simulink model "DBX_control_harness"  (R2015a)
settings: Solver=ode2  SolverMode=SingleTasking  StartTime=0.0  StopTime=inf  FixedStep=T_sim  RelTol=1e-3
values from neighbouring files (symbols this model uses):
  airport_alt = 587.5    [Run_DBX.m]
  latitude = 40.463650    (= 40.46365)    [Run_DBX.m]
  longitude = -3.554389    [Run_DBX.m]
  T_ctrl = 0.01    [Run_DBX.m]
  T_sim = 0.01    [Run_DBX.m]
undefined symbols (not defined in the file or in its folder): accel_sigmas, Alt_0, DBX_PWM, delta_a_L_0_servo, delta_a_R_0_servo, delta_rv_L_0_servo, delta_rv_R_0_servo, eta_1_0_servo, eta_2_0_servo, eta_3_0_servo, Euler_0, Euler_dot_sigmas, Euler_sigmas, g, GPS_pos_sig, Initial_Omegas, Newton, omgea_b_sigmas, qbar_sigma, quaternion_sigmas, Raphson, Roll_pich_sens, sigbuilder_block, Speed_sigmas, TAS_0, tau_1_0, tau_2_0, tau_3_0, Throtle_sens, Volt_noise, Yaw_sens
libraries: DBX_model x14, commnoisgen2 x9, simulink x3, powerlib_meascontrol x2, utility x1
(part 1 of 2)
settings Model: ExtModeTrigDuration=5000  Creator=DavidTorres  LastModifiedBy=david
settings DataIOCC: LimitDataPoints=off  SaveOutput=off  SignalLogging=off  DSMLogging=off  VisualizeSimOutput=off  SaveTime=off
settings OptimizationCC: InlineParams=on  UseDivisionForNetSlopeComputation=on  UseFloatMulNetSlope=on  InlineInvariantSignals=on  EnhancedBackFolding=on  EfficientFloat2IntCast=on  MaxStackSize=inf  SimCompilerOptimization=on
settings DebuggingCC: WriteAfterWriteMsg=EnableAllAsError  AlgebraicLoopMsg=error  ArtificialAlgebraicLoopMsg=error  SaveWithParameterizedLinksMsg=none  IntegerOverflowMsg=error  ParameterUnderflowMsg=error  ParameterTunabilityLossMsg=error  UniqueDataStoreMsg=error  AssertControl=DisableAll  StrictBusMsg=ErrorOnBusTreatedAsVector  NonBusSignalsTreatedAsBus=error  SFUnexpectedBacktrackingDiag=error  SFInvalidInputDataAccessInChartInitDiag=error  SFNoUnconditionalDefaultTransitionDiag=error  SFTransitionOutsideNaturalParentDiag=error  SFUnconditionalTransitionShadowingDiag=error  SFUndirectedBroadcastEventsDiag=error  SFTransitionActionBeforeConditionDiag=error  IntegerSaturationMsg=error
settings HardwareCC: ProdLargestAtomicInteger=Long  ProdLargestAtomicFloat=Float  ProdIntDivRoundTo=Zero  ProdEndianess=LittleEndian  ProdHWDeviceType=ARM Compatible->ARM 7  TargetUnknown=on
settings ModelReferenceCC: ModelReferenceNumInstancesAllowed=Single  ModelReferencePassRootInputsByReference=off

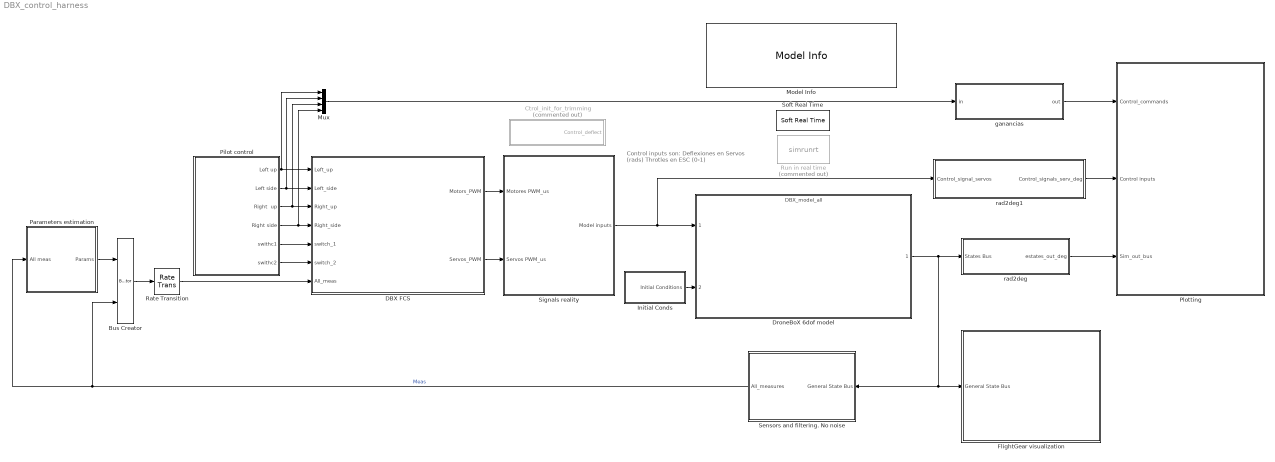
== system DBX_control_harness ==
  note: Control inputs son:
      | Deflexiones en Servos (rads)
      | Throtles en ESC (0-1)
  Bus Creator : BusCreator  Inputs=2
  Ctrol_init_for_trimming : Subsystem  Commented=on  TreatAsAtomicUnit=on
  DBX FCS : Subsystem
  DroneBoX 6dof model : ModelReference  ModelNameDialog=DBX_model_all.slx  SimulationMode=Normal  OverrideUsingVariant=Model_all  ModelReferenceVersion=1.02  CopyOfModelName=DBX_model_all.slx  DefaultDataLogging=on
      mask Display:
      | % % image('conv.jpg')
      | % %
      | % % port_label('output', 1, 'General State Bus')
      | % %
      | % % port_label('input', 1, 'Control Inputs')
      | % % port_label('input', 2, 'Initial Conditions')
      | % %
      | % %
      | % % % Variant dealing
      | % % ActiveVar = get_param(gcb,'activevariant');
      | % % disp(['{\bf\fontsize{16}',ActiveVar,'}'], 'texmode','on');
  FlightGear visualization : Subsystem  TreatAsAtomicUnit=on
      mask Display:
      | % % disp('{\bf\fontsize{20} Flight Gear}', 'texmode','on');
      | % % image('convFG.jpg')
      | % %
      | % % port_label('input', 1, 'General State Bus')
  Initial Conds : Subsystem  TreatAsAtomicUnit=on
  Model Info : simulink/Model-Wide Utilities/Model Info  Frame=on  DisplayStringWithTags=|  HorizontalTextAlignment=Center  LeftAlignmentValue=0.5  SourceBlockDiagram=DBX_control_harness  TagMaxNumber=20
      | Model %<ModelName>
      | 
      | Creado por %<Creator>
      | Modificado el %<LastModificationDate> por %<LastModifiedBy>
      | Version %<ModelVersion>
  Mux : Mux
  Parameters estimation : Subsystem  TreatAsAtomicUnit=on
  "Pilot control " : Subsystem  Variant=on  OverrideUsingVariant=Turnigy
  Plotting : Subsystem
      mask Display:
      | disp('{\bf\fontsize{20} Plotting}', 'texmode','on');
      | % port_label('input', 1, 'States')
      | % port_label('input', 2, 'Demans')
  Rate Transition : RateTransition  OutPortSampleTime=T_ctrl
  Run in real time : S-Function  Commented=on  FunctionName=simrunrt  Parameters=1
  Sensors and filtering. No noise : Subsystem  Variant=on  VariantControl=No noise  OverrideUsingVariant=Noise
  Signals reality : Subsystem
  Soft Real Time : utility/Soft Real Time  x=1
  ganancias : Subsystem
  rad2deg : Subsystem
  rad2deg1 : Subsystem
  wires:
  Initial Conds/1(Initial Conditions) -> DroneBoX 6dof model/2
  DroneBoX 6dof model/1 -> FlightGear visualization/1(General State Bus), Sensors and filtering. No noise/1(General State Bus), rad2deg/1(States Bus)
  rad2deg/1("estates_out_deg ") -> Plotting/3(Sim_out_bus)
  Signals reality/1(Model inputs) -> rad2deg1/1(Control_signal_servos), DroneBoX 6dof model/1
  Sensors and filtering. No noise/1(All_measures) -> Parameters estimation/1(All meas), Bus Creator/2  "Meas"
  Bus Creator/1 -> Rate Transition/1
  Parameters estimation/1(Params) -> Bus Creator/1
  DBX FCS/1(Motors_PWM) -> Signals reality/1(Motores PWM_us)
  DBX FCS/2(Servos_PWM) -> Signals reality/2(Servos PWM_us)
  Rate Transition/1 -> DBX FCS/7(All_meas)
  rad2deg1/1("Control_signals_serv_deg ") -> Plotting/2(Control inputs)
  "Pilot control "/1(Left up) -> DBX FCS/1(Left_up), Mux/1
  "Pilot control "/2(Left side) -> DBX FCS/2(Left_side), Mux/2
  "Pilot control "/3(Right  up) -> DBX FCS/3(Right_up), Mux/3
  Mux/1 -> ganancias/1(in)
  ganancias/1(out) -> Plotting/1(Control_commands)
  "Pilot control "/6(swithc2) -> DBX FCS/6(switch_2)
  "Pilot control "/5(swithc1) -> DBX FCS/5(switch_1)
  "Pilot control "/4(Right side) -> DBX FCS/4(Right_side), Mux/4

== system DBX_control_harness/Ctrol_init_for_trimming ==
  note: Control inputs (servos angles):
      | 1. tau_1 [0-1] (Thr ottle motor 1)
      | 2. eta_1 (rad)  (Pan arm 1)
      |
      | 3. tau_2 [0-1] (Throttle motor 2)
      | 4. eta_2 (rad)  (Pan arm 2)
      |
      | 5. tau_3 [0-1] (Throttle motor 3)
      | 6. eta_3 (rad)  (Pan arm  3)
      |
      | 7. Rudervator Left (rad)
      | 8. Rudervator Right (rad)
      | 9. Aileron Left (rad)
      | 10. Aielron Right (rad)
  Constant : Constant  Value=[tau_1_0,eta_1_0_servo,tau_2_0,eta_2_0_servo,tau_3_0,eta_3_0_servo,delta_rv_L_0_servo,delta_rv_R_0_servo,delta_a_L_0_servo,delta_a_R_0_servo]'
  Control_deflect : Outport
  wires:
  Constant/1 -> Control_deflect/1

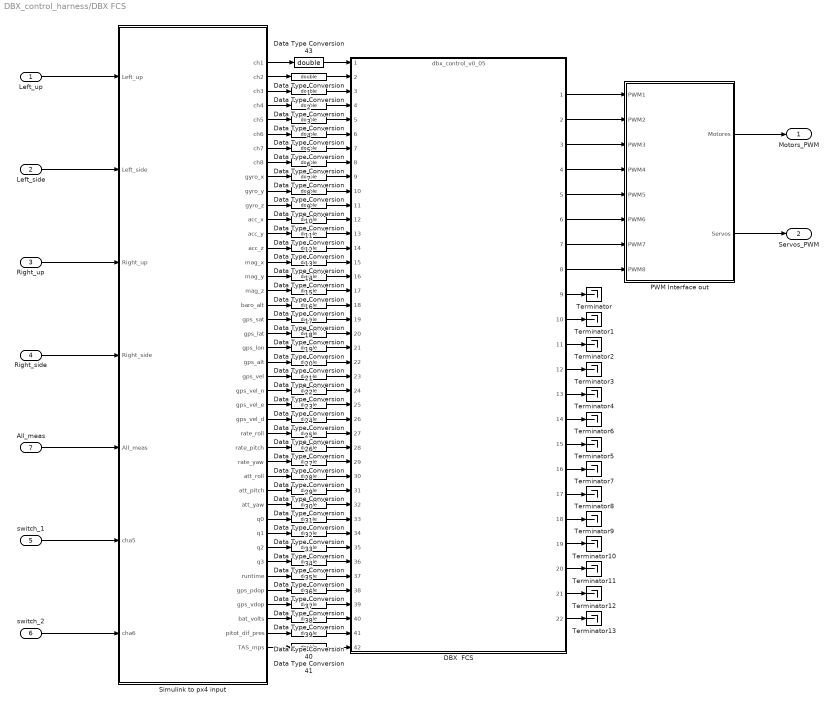
== system DBX_control_harness/DBX FCS ==
  Left_up : Inport
  Left_side : Inport  Port=2
  Right_up : Inport  Port=3
  Right_side : Inport  Port=4
  switch_1 : Inport  Port=5
  switch_2 : Inport  Port=6
  All_meas : Inport  Port=7
  DBX  FCS : ModelReference  ModelNameDialog=dbx_control_v0_05.slx  ModelReferenceVersion=0.05  CopyOfModelName=dbx_control_v0_05.slx  DefaultDataLogging=on
  Data Type Conversion{1..41,43} (42 alike) : DataTypeConversion  OutDataTypeStr=double
  PWM Interface out : Subsystem  Variant=on  VariantControl=Variant1  OverrideUsingVariant=Octubre
  Simulink to px4 input : Subsystem  TreatAsAtomicUnit=on
  Terminator{,1..13} (14 alike) : Terminator
  Motors_PWM : Outport
  Servos_PWM : Outport  Port=2
  wires:
  PWM Interface out/1(Motores) -> Motors_PWM/1
  PWM Interface out/2(Servos) -> Servos_PWM/1
  Left_up/1 -> Simulink to px4 input/1(Left_up)
  Left_side/1 -> Simulink to px4 input/2(Left_side)
  Right_up/1 -> Simulink to px4 input/3(Right_up)
  Right_side/1 -> Simulink to px4 input/4(Right_side)
  All_meas/1 -> Simulink to px4 input/5(All_meas)
  switch_2/1 -> Simulink to px4 input/7(cha6)
  switch_1/1 -> Simulink to px4 input/6(cha5)
  Simulink to px4 input/24(gps_vel_n) -> Data Type Conversion23/1
  Simulink to px4 input/25(gps_vel_e) -> Data Type Conversion24/1
  Simulink to px4 input/26(gps_vel_d) -> Data Type Conversion25/1
  Simulink to px4 input/27(rate_roll) -> Data Type Conversion26/1
  Simulink to px4 input/28(rate_pitch) -> Data Type Conversion27/1
  Simulink to px4 input/29(rate_yaw) -> Data Type Conversion28/1
  Simulink to px4 input/30(att_roll) -> Data Type Conversion29/1
  Simulink to px4 input/31(att_pitch) -> Data Type Conversion30/1
  Simulink to px4 input/32(att_yaw) -> Data Type Conversion31/1
  Simulink to px4 input/33(q0) -> Data Type Conversion32/1
  Simulink to px4 input/34(q1) -> Data Type Conversion33/1
  Simulink to px4 input/10(gyro_y) -> Data Type Conversion9/1
  Simulink to px4 input/11(gyro_z) -> Data Type Conversion10/1
  Simulink to px4 input/12(acc_x) -> Data Type Conversion11/1
  Simulink to px4 input/13(acc_y) -> Data Type Conversion12/1
  Simulink to px4 input/14(acc_z) -> Data Type Conversion13/1
  Simulink to px4 input/15(mag_x) -> Data Type Conversion14/1
  Simulink to px4 input/16(mag_y) -> Data Type Conversion15/1
  Simulink to px4 input/17(mag_z) -> Data Type Conversion16/1
  Simulink to px4 input/18(baro_alt) -> Data Type Conversion17/1
  Simulink to px4 input/19(gps_sat) -> Data Type Conversion18/1
  Simulink to px4 input/20(gps_lat) -> Data Type Conversion19/1
  Simulink to px4 input/21(gps_lon) -> Data Type Conversion20/1
  Simulink to px4 input/22(gps_alt) -> Data Type Conversion21/1
  Simulink to px4 input/23(gps_vel) -> Data Type Conversion22/1
  Simulink to px4 input/35(q2) -> Data Type Conversion34/1
  Simulink to px4 input/36(q3) -> Data Type Conversion35/1
  Simulink to px4 input/37(runtime) -> Data Type Conversion36/1
  Simulink to px4 input/38(gps_pdop) -> Data Type Conversion37/1
  Simulink to px4 input/39(gps_vdop) -> Data Type Conversion38/1
  Simulink to px4 input/40(bat_volts) -> Data Type Conversion39/1
  Simulink to px4 input/1(ch1) -> Data Type Conversion43/1
  Simulink to px4 input/2(ch2) -> Data Type Conversion1/1
  Simulink to px4 input/3(ch3) -> Data Type Conversion2/1
  Simulink to px4 input/4(ch4) -> Data Type Conversion3/1
  Simulink to px4 input/5(ch5) -> Data Type Conversion4/1
  Simulink to px4 input/6(ch6) -> Data Type Conversion5/1
  Simulink to px4 input/7(ch7) -> Data Type Conversion6/1
  Simulink to px4 input/8(ch8) -> Data Type Conversion7/1
  Simulink to px4 input/9(gyro_x) -> Data Type Conversion8/1
  Simulink to px4 input/41(pitot_dif_pres) -> Data Type Conversion40/1
  DBX  FCS/1 -> PWM Interface out/1(PWM1)
  DBX  FCS/2 -> PWM Interface out/2(PWM2)
  DBX  FCS/3 -> PWM Interface out/3(PWM3)
  DBX  FCS/4 -> PWM Interface out/4(PWM4)
  DBX  FCS/5 -> PWM Interface out/5(PWM5)
  DBX  FCS/6 -> PWM Interface out/6(PWM6)
  DBX  FCS/7 -> PWM Interface out/7(PWM7)
  DBX  FCS/8 -> PWM Interface out/8(PWM8)
  Simulink to px4 input/42(TAS_mps) -> Data Type Conversion41/1
  DBX  FCS/9 -> Terminator/1
  DBX  FCS/10 -> Terminator1/1
  DBX  FCS/11 -> Terminator2/1
  DBX  FCS/12 -> Terminator3/1
  DBX  FCS/15 -> Terminator5/1
  DBX  FCS/14 -> Terminator6/1
  DBX  FCS/13 -> Terminator4/1
  DBX  FCS/16 -> Terminator7/1
  DBX  FCS/17 -> Terminator8/1
  DBX  FCS/18 -> Terminator9/1
  DBX  FCS/19 -> Terminator10/1
  DBX  FCS/20 -> Terminator11/1
  DBX  FCS/21 -> Terminator12/1
  DBX  FCS/22 -> Terminator13/1
  Data Type Conversion43/1 -> DBX  FCS/1
  Data Type Conversion1/1 -> DBX  FCS/2
  Data Type Conversion2/1 -> DBX  FCS/3
  Data Type Conversion3/1 -> DBX  FCS/4
  Data Type Conversion4/1 -> DBX  FCS/5
  Data Type Conversion5/1 -> DBX  FCS/6
  Data Type Conversion6/1 -> DBX  FCS/7
  Data Type Conversion7/1 -> DBX  FCS/8
  Data Type Conversion8/1 -> DBX  FCS/9
  Data Type Conversion9/1 -> DBX  FCS/10
  Data Type Conversion10/1 -> DBX  FCS/11
  Data Type Conversion11/1 -> DBX  FCS/12
  Data Type Conversion12/1 -> DBX  FCS/13
  Data Type Conversion13/1 -> DBX  FCS/14
  Data Type Conversion14/1 -> DBX  FCS/15
  Data Type Conversion15/1 -> DBX  FCS/16
  Data Type Conversion16/1 -> DBX  FCS/17
  Data Type Conversion17/1 -> DBX  FCS/18
  Data Type Conversion18/1 -> DBX  FCS/19
  Data Type Conversion19/1 -> DBX  FCS/20
  Data Type Conversion20/1 -> DBX  FCS/21
  Data Type Conversion21/1 -> DBX  FCS/22
  Data Type Conversion22/1 -> DBX  FCS/23
  Data Type Conversion23/1 -> DBX  FCS/24
  Data Type Conversion24/1 -> DBX  FCS/25
  Data Type Conversion25/1 -> DBX  FCS/26
  Data Type Conversion26/1 -> DBX  FCS/27
  Data Type Conversion27/1 -> DBX  FCS/28
  Data Type Conversion28/1 -> DBX  FCS/29
  Data Type Conversion29/1 -> DBX  FCS/30
  Data Type Conversion30/1 -> DBX  FCS/31
  Data Type Conversion31/1 -> DBX  FCS/32
  Data Type Conversion32/1 -> DBX  FCS/33
  Data Type Conversion33/1 -> DBX  FCS/34
  Data Type Conversion34/1 -> DBX  FCS/35
  Data Type Conversion35/1 -> DBX  FCS/36
  Data Type Conversion36/1 -> DBX  FCS/37
  Data Type Conversion37/1 -> DBX  FCS/38
  Data Type Conversion38/1 -> DBX  FCS/39
  Data Type Conversion39/1 -> DBX  FCS/40
  Data Type Conversion40/1 -> DBX  FCS/41
  Data Type Conversion41/1 -> DBX  FCS/42

== system DBX_control_harness/FlightGear visualization ==
  General State Bus : Inport
  Bus Selector1 : BusSelector  OutputSignals=euler
  Bus Selector4 : BusSelector  OutputSignals=X_e
  Demux : Demux  Outputs=3
  Flat Earth to LLA : Subsystem
  Mux : Mux  Inputs=6
  Saturation : Saturate  UpperLimit=1e8  LowerLimit=-1e5  OutDataTypeStr=double
  Send2FG : S-Function  FunctionName=sim2fg  Parameters='localhost',5502
  cast1 : DataTypeConversion  OutDataTypeStr=double  SaturateOnIntegerOverflow=on
  href : Constant  Value=airport_alt  VectorParams1D=off
  keep pi/pi : Subsystem
  wires:
  Demux/2 -> Mux/5
  Demux/1 -> Mux/4
  href/1 -> Flat Earth to LLA/2(altitude0)
  General State Bus/1 -> Bus Selector1/1, Bus Selector4/1
  Bus Selector1/1 -> keep pi/pi/1(phi theta psi)  "<euler>"
  Saturation/1 -> Mux/3
  Bus Selector4/1 -> Flat Earth to LLA/1(Xe)  "<X_e>"
  Mux/1 -> cast1/1
  cast1/1 -> Send2FG/1
  keep pi/pi/1(ptp_earth) -> Demux/1
  Demux/3 -> Mux/6
  Flat Earth to LLA/3(altitude h) -> Saturation/1
  Flat Earth to LLA/2(latitude mu) -> Mux/1
  Flat Earth to LLA/1(longitude l) -> Mux/2

== system DBX_control_harness/Initial Conds ==
  Bus Creator : BusCreator  Inputs=5  OutDataTypeStr=Bus: slBus1
  Ini Position X_e_0 : Constant  Value=[0;0;-Alt_0]
  Initial Attitude Euler_0 : Constant  Value=Euler_0
  Initial Attitude Rate  Euler_dot_0 : Constant  Value=[deg2rad(0);deg2rad(0);deg2rad(0)]
  Initial Velocity V_e_0 : Constant  Value=[TAS_0;0;0]
  Initial omegas : Constant  Value=Initial_Omegas
  Initial Conditions : Outport
  wires:
  Ini Position X_e_0/1 -> Bus Creator/1  "X_e_0"
  Initial Velocity V_e_0/1 -> Bus Creator/2  "V_e_0"
  Initial Attitude Euler_0/1 -> Bus Creator/3  "Euler_0"
  Initial Attitude Rate  Euler_dot_0/1 -> Bus Creator/4  "Euler_dot_0"
  Bus Creator/1 -> Initial Conditions/1
  Initial omegas/1 -> Bus Creator/5  "Init_Omegas"

== system DBX_control_harness/Parameters estimation ==
  note: This is T_Fb->Fe
  All meas : Inport
  Bus Creator : BusCreator  Inputs=8
  Bus Selector : BusSelector  OutputSignals=A_accel meas,Euler meas (rad),V_e_meas
  DCM1 : Subsystem  TreatAsAtomicUnit=on
  Dot Product : DotProduct  InputSameDT=on  OutDataTypeStr=Inherit: Inherit via internal rule
  GPS_sat : Constant  Value=5
  MATLAB Function : MATLAB Function  TreatAsAtomicUnit=on
  Matrix Multiply1 : Product  Multiplication=Matrix(*)
  Matrix Multiply2 : Product  Multiplication=Matrix(*)
  Permute Dimensions : PermuteDimensions
  Selector1 : Selector  InputPortWidth=3  Indices=3
  Selector7 : Selector  InputPortWidth=3  Indices=[3 2 1]
  Sqrt : Sqrt  SaturateOnIntegerOverflow=on
  Sum : Sum  Inputs=+-|
  g : Constant  Value=[0;0;g]
  gps_vdop : Constant  Value=1.5
  p_dop : Constant  Value=1.5
  Params : Outport
  wires:
  All meas/1 -> Bus Selector/1
  Bus Selector/2 -> Selector1/1, Selector7/1  "<Euler meas (rad)>"
  DCM1/1(DCM) -> Permute Dimensions/1, Bus Creator/2  "DCM"
  Selector7/1 -> DCM1/1(Euler)
  Bus Creator/1 -> Params/1  "Params"
  Selector1/1 -> MATLAB Function/1(yaw)
  MATLAB Function/1(T_yaw) -> Matrix Multiply2/1, Bus Creator/3  "T_Fe-Fyaw"
  Matrix Multiply2/1 -> Bus Creator/4  "V_yaw"
  Bus Selector/3 -> Dot Product/1, Dot Product/2, Matrix Multiply2/2  "<V_e_meas>"
  Permute Dimensions/1 -> Matrix Multiply1/1
  g/1 -> Matrix Multiply1/2
  Matrix Multiply1/1 -> Sum/2
  Bus Selector/1 -> Sum/1  "<A_accel meas>"
  Sum/1 -> Bus Creator/1  "a_meas"
  p_dop/1 -> Bus Creator/5  "gps_pdop"
  GPS_sat/1 -> Bus Creator/7  "gps_sat"
  gps_vdop/1 -> Bus Creator/6  "gps_vdop"
  Sqrt/1 -> Bus Creator/8  "TAS_mps"
  Dot Product/1 -> Sqrt/1

== system DBX_control_harness/Pilot control  ==
  "Logitec " : Subsystem  VariantControl=Logitec
  Signal generator : Subsystem  VariantControl=Signal_gen
  Turnigy TX (XTR G2 FMS) : Subsystem  VariantControl=Turnigy
  Left up : Outport
  Left side : Outport  Port=2
  Right  up : Outport  Port=3
  Right side : Outport  Port=4
  swithc1 : Outport  Port=5
  swithc2 : Outport  Port=6

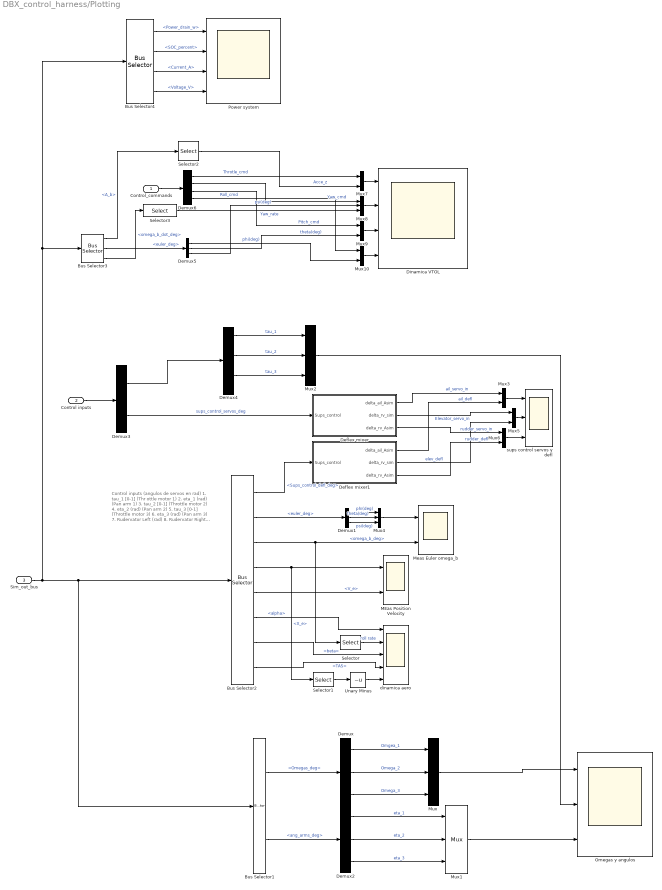
== system DBX_control_harness/Plotting ==
  note: Control inputs (angulos de servos en rad)
      | 1. tau_1 [0-1] (Thr ottle motor 1)
      | 2. eta_1 (rad)  (Pan arm 1)
      |
      | 3. tau_2 [0-1] (Throttle motor 2)
      | 4. eta_2 (rad)  (Pan arm 2)
      |
      | 5. tau_3 [0-1] (Throttle motor 3)
      | 6. eta_3 (rad)  (Pan arm  3)
      |
      | 7. Rudervator Left (rad)
      | 8. Rudervator Right (rad)
      | 9. Aileron Left (rad)
      | 10. Aielron Right (rad)
  Control_commands : Inport
  Control inputs : Inport  Port=2
  Sim_out_bus : Inport  Port=3
  Bus Selector1 : BusSelector  OutputSignals=Omegas_deg,ang_arms_deg
  Bus Selector2 : BusSelector  OutputSignals=Sups_control_defl_deg,euler_deg,omega_b_deg,X_e,V_e,Aero_vars.alpha,Aero_vars.beta,Aero_vars.TAS
  Bus Selector3 : BusSelector  OutputSignals=A_b,euler_deg,omega_b_dot_deg
  Bus Selector4 : BusSelector  OutputSignals=Power_drain_w,Battery_bus.SOC_percent,Battery_bus.Current_A,Battery_bus.Voltage_V
  Deflex mixer : Subsystem  TreatAsAtomicUnit=on
  Deflex mixer1 : Subsystem  TreatAsAtomicUnit=on
  Demux{,1..2,5} (4 alike) : Demux  Outputs=3
  Demux3 : Demux  Outputs=[6,4]
  Demux4 : Demux  Outputs=6
  Demux6 : Demux
  Dinamica VTOL : Scope  NumInputPorts=4
      settings: ShowLegends=on  TimeRange=50  YMin=-3~-200~-8~-5  YMax=5~100~4~10  SaveName=ScopeData5
  MEas Position Velocity : Scope  NumInputPorts=2
      settings: ShowLegends=on  TimeRange=100  YMin=-35~-5  YMax=10~6  SaveName=ScopeData3
  Meas Euler omega_b : Scope  NumInputPorts=2
      settings: ShowLegends=on  TimeRange=50  YMin=-15~-25  YMax=20~25  SaveName=ScopeData4
  Mux{,1..2,4,8} (5 alike) : Mux  Inputs=3
  Mux{3,5..7,9..10} (6 alike) : Mux  Inputs=2
  Omegas y angulos : Scope  NumInputPorts=3
      settings: ShowLegends=on  TimeRange=50  YMin=0~0~-100  YMax=37500~0.5~0
  Power system : Scope  NumInputPorts=4
      settings: ShowLegends=on  TimeRange=300  YMin=460~55~54~29  YMax=580~61~58~29.225  SaveName=ScopeData6
  Selector : Selector  InputPortWidth=3
  Selector1 : Selector  InputPortWidth=3  Indices=3
  Selector2 : Selector  InputPortWidth=3
  Selector3 : Selector  InputPortWidth=3  Indices=3
  Unary Minus : UnaryMinus
  dinamica aero : Scope  NumInputPorts=5
      settings: ShowLegends=on  TimeRange=100  YMin=-3~-10~-0.75~17.5~20  YMax=6~17.5~0.75~32.5~45
  sups control servos y defl : Scope  NumInputPorts=3
      settings: ShowLegends=on  TimeRange=100  YMin=-1~-8~-1  YMax=1~-5~1  SaveName=ScopeData2
  wires:
  Bus Selector2/2 -> Demux1/1  "<euler_deg>"
  Bus Selector2/4 -> MEas Position Velocity/1, Selector1/1  "<X_e>"
  Demux1/3 -> Mux4/3  "psi(deg)"
  Demux1/1 -> Mux4/1  "phi(deg)"
  Demux1/2 -> Mux4/2  "theta(deg)"
  Mux4/1 -> Meas Euler omega_b/1
  Bus Selector2/3 -> Selector/1, Meas Euler omega_b/2  "<omega_b_deg>"
  Bus Selector2/5 -> MEas Position Velocity/2  "<V_e>"
  Sim_out_bus/1 -> Bus Selector4/1, Bus Selector3/1, Bus Selector2/1, Bus Selector1/1
  Bus Selector1/1 -> Demux/1  "<Omegas_deg>"
  Bus Selector1/2 -> Demux2/1  "<ang_arms_deg>"
  Demux/1 -> Mux/1  "Omgea_1"
  Demux2/1 -> Mux1/1  "eta_1"
  Demux/2 -> Mux/2  "Omega_2"
  Demux2/2 -> Mux1/2  "eta_2"
  Demux/3 -> Mux/3  "Omega_3"
  Demux2/3 -> Mux1/3  "eta_3"
  Control inputs/1 -> Demux3/1
  Bus Selector2/6 -> dinamica aero/1  "<alpha>"
  Bus Selector2/7 -> dinamica aero/3  "<beta>"
  Bus Selector2/8 -> dinamica aero/4  "<TAS>"
  Selector/1 -> dinamica aero/2  "roll rate"
  Demux3/2 -> Deflex mixer/1(Sups_control)  "sups_control_servos_deg"
  Demux3/1 -> Demux4/1
  Demux4/1 -> Mux2/1  "tau_1"
  Demux4/3 -> Mux2/2  "tau_2"
  Demux4/5 -> Mux2/3  "tau_3"
  Mux2/1 -> Omegas y angulos/2
  Mux/1 -> Omegas y angulos/1
  Mux1/1 -> Omegas y angulos/3
  Selector1/1 -> Unary Minus/1
  Unary Minus/1 -> dinamica aero/5
  Bus Selector2/1 -> Deflex mixer1/1(Sups_control)  "<Sups_control_defl_deg>"
  Mux3/1 -> sups control servos y defl/1
  Deflex mixer1/1(delta_ail_Asim) -> Mux3/2  "ail_defl"
  Deflex mixer/1(delta_ail_Asim) -> Mux3/1  "ail_servo_in"
  Mux5/1 -> sups control servos y defl/2
  Deflex mixer/2(delta_rv_sim) -> Mux5/1  "Elevator_servo_in"
  Deflex mixer1/2(delta_rv_sim) -> Mux5/2  "elev_defl"
  Mux6/1 -> sups control servos y defl/3
  Deflex mixer/3(delta_rv_Asim) -> Mux6/1  "rudder_servo_in"
  Deflex mixer1/3(delta_rv_Asim) -> Mux6/2  "rudder_defl"
  Bus Selector3/2 -> Demux5/1  "<euler_deg>"
  Demux5/3 -> Mux8/2  "psi(deg)"
  Demux5/1 -> Mux10/2  "phi(deg)"
  Demux5/2 -> Mux9/2  "theta(deg)"
  Control_commands/1 -> Demux6/1
  Demux6/1 -> Mux7/1  "Throtle_cmd"
  Bus Selector3/1 -> Selector2/1  "<A_b>"
  Selector2/1 -> Mux7/2  "Acce_z"
  Demux6/2 -> Mux8/1  "Yaw_cmd"
  Bus Selector3/3 -> Selector3/1  "<omega_b_dot_deg>"
  Selector3/1 -> Mux8/3  "Yaw_rate"
  Demux6/3 -> Mux9/1  "Pitch_cmd"
  Demux6/4 -> Mux10/1  "Roll_cmd"
  Mux7/1 -> Dinamica VTOL/1
  Mux8/1 -> Dinamica VTOL/2
  Mux9/1 -> Dinamica VTOL/3
  Mux10/1 -> Dinamica VTOL/4
  Bus Selector4/3 -> Power system/3  "<Current_A>"
  Bus Selector4/4 -> Power system/4  "<Voltage_V>"
  Bus Selector4/1 -> Power system/1  "<Power_drain_w>"
  Bus Selector4/2 -> Power system/2  "<SOC_percent>"

== system DBX_control_harness/Sensors and filtering. No noise ==
  General State Bus : Inport
  Sensors and filtering. NOISE : Subsystem  VariantControl=Noise
  Sensors and filtering. No noise : Subsystem  VariantControl=No_noise
  All_measures : Outport

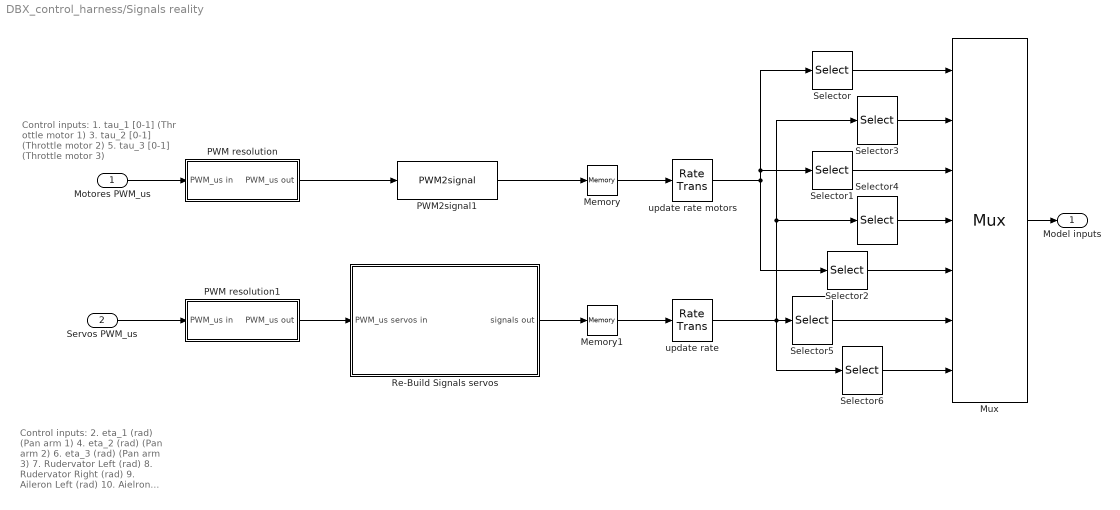
== system DBX_control_harness/Signals reality ==
  note: Control inputs:
      | 1. tau_1 [0-1] (Thr ottle motor 1)
      |
      | 3. tau_2 [0-1] (Throttle motor 2)
      |
      | 5. tau_3 [0-1] (Throttle motor 3)
  note: Control inputs:
      | 2. eta_1 (rad)  (Pan arm 1)
      |
      | 4. eta_2 (rad)  (Pan arm 2)
      |
      | 6. eta_3 (rad)  (Pan arm  3)
      |
      | 7. Rudervator Left (rad)
      | 8. Rudervator Right (rad)
      | 9. Aileron Left (rad)
      | 10. Aielron Right (rad)
  Motores PWM_us : Inport
  Servos PWM_us : Inport  Port=2
  Memory : Memory  X0=[tau_1_0,tau_2_0,tau_3_0]'  InheritSampleTime=on
  Memory1 : Memory  X0=[eta_1_0_servo,eta_3_0_servo,eta_3_0_servo,delta_rv_L_0_servo,delta_rv_R_0_servo,delta_a_L_0_servo,delta_a_R_0_servo]'  InheritSampleTime=on
  Mux : Mux  Inputs=[1,1,1,1,1,1,4]
  PWM resolution : Subsystem  TreatAsAtomicUnit=on
  PWM resolution1 : Subsystem  TreatAsAtomicUnit=on
  PWM2signal1 : DBX_model/PWM2signal  c=DBX_PWM.Motors.Max_PWM  a=DBX_PWM.Motors.Min_PWM  d=1  b=0
  Re-Build Signals servos : Subsystem  TreatAsAtomicUnit=on
  Selector : Selector  InputPortWidth=3
  Selector1 : Selector  InputPortWidth=3  Indices=2
  Selector2 : Selector  InputPortWidth=3  Indices=3
  Selector3 : Selector  InputPortWidth=7  Indices=[1]
  Selector4 : Selector  InputPortWidth=7  Indices=2
  Selector5 : Selector  InputPortWidth=7  Indices=3
  Selector6 : Selector  InputPortWidth=7  Indices=[4:7]
  update rate : RateTransition  OutPortSampleTime=1/DBX_PWM.Servos.update_rate
  update rate motors : RateTransition  OutPortSampleTime=1/DBX_PWM.Motors.update_rate
  Model inputs : Outport
  wires:
  Motores PWM_us/1 -> PWM resolution/1(PWM_us in)
  Memory/1 -> update rate motors/1
  PWM resolution/1(PWM_us out) -> PWM2signal1/1
  Servos PWM_us/1 -> PWM resolution1/1(PWM_us in)
  Re-Build Signals servos/1(signals out) -> Memory1/1
  PWM resolution1/1(PWM_us out) -> Re-Build Signals servos/1(PWM_us servos in)
  Memory1/1 -> update rate/1
  Mux/1 -> Model inputs/1
  update rate motors/1 -> Selector1/1, Selector/1, Selector2/1
  Selector/1 -> Mux/1
  update rate/1 -> Selector6/1, Selector5/1, Selector4/1, Selector3/1
  Selector3/1 -> Mux/2
  PWM2signal1/1 -> Memory/1
  Selector1/1 -> Mux/3
  Selector4/1 -> Mux/4
  Selector2/1 -> Mux/5
  Selector5/1 -> Mux/6
  Selector6/1 -> Mux/7

== system DBX_control_harness/ganancias ==
  in : Inport
  Demux : Demux
  Mux : Mux
  r2d1 : Gain  Gain=Throtle_sens
  r2d2 : Gain  Gain=Yaw_sens
  r2d3 : Gain  Gain=-Roll_pich_sens
  r2d4 : Gain  Gain=Roll_pich_sens
  out : Outport
  wires:
  Mux/1 -> out/1
  in/1 -> Demux/1
  Demux/1 -> r2d1/1
  Demux/2 -> r2d2/1
  Demux/4 -> r2d4/1
  Demux/3 -> r2d3/1
  r2d1/1 -> Mux/1
  r2d2/1 -> Mux/2
  r2d3/1 -> Mux/3
  r2d4/1 -> Mux/4

== system DBX_control_harness/rad2deg ==
  States Bus : Inport
  Bus Creator : BusCreator  Inputs=17
  Bus Creator1 : BusCreator  Inputs=3
  Bus Selector2 : BusSelector  OutputSignals=X_e,V_e,V_b,omega_b,q,omega_dot,A_b,DCM_Vect,euler,euler_dot,A_s,Omegas,Ang_arms_rad,Aero_vars.TAS,Aero_vars.beta,Aero_vars.alpha,Sups_control_defl,Battery_bus,Power_drain_w
  Bus to Vector : BusToVector
  r2d{,1..8} (9 alike) : Gain  Gain=180/pi
  "estates_out_deg " : Outport
  wires:
  States Bus/1 -> Bus Selector2/1
  Bus Selector2/2 -> Bus Creator/2  "<V_e>"
  Bus Selector2/3 -> Bus Creator/3  "<V_b>"
  Bus Selector2/4 -> r2d/1  "<omega_b>"
  Bus Selector2/5 -> Bus Creator/5  "<q>"
  Bus Selector2/6 -> r2d1/1  "<omega_dot>"
  Bus Selector2/7 -> Bus Creator/7  "<A_b>"
  Bus Selector2/8 -> Bus Creator/8  "<DCM_Vect>"
  Bus Selector2/9 -> r2d2/1  "<euler>"
  Bus Selector2/10 -> r2d3/1  "<euler_dot>"
  Bus Selector2/11 -> Bus Creator/11  "<A_s>"
  Bus Selector2/12 -> r2d4/1  "<Omegas>"
  Bus Selector2/13 -> Bus to Vector/1  "<Ang_arms_rad>"
  Bus Selector2/1 -> Bus Creator/1  "<X_e>"
  r2d/1 -> Bus Creator/4  "omega_b_deg"
  r2d1/1 -> Bus Creator/6  "omega_b_dot_deg"
  r2d2/1 -> Bus Creator/9  "euler_deg"
  r2d3/1 -> Bus Creator/10  "euler_dot_deg"
  r2d4/1 -> Bus Creator/12  "Omegas_deg"
  r2d5/1 -> Bus Creator/13  "ang_arms_deg"
  Bus Creator/1 -> "estates_out_deg "/1
  Bus to Vector/1 -> r2d5/1
  Bus Selector2/14 -> Bus Creator1/1  "<TAS>"
  Bus Selector2/15 -> r2d6/1  "<beta>"
  Bus Creator1/1 -> Bus Creator/14  "Aero_vars"
  r2d6/1 -> Bus Creator1/2  "beta"
  r2d7/1 -> Bus Creator1/3  "alpha"
  r2d8/1 -> Bus Creator/15  "Sups_control_defl_deg"
  Bus Selector2/17 -> r2d8/1  "<Sups_control_defl>"
  Bus Selector2/16 -> r2d7/1  "<alpha>"
  Bus Selector2/19 -> Bus Creator/17  "<Power_drain_w>"
  Bus Selector2/18 -> Bus Creator/16  "<Battery_bus>"

== system DBX_control_harness/rad2deg1 ==
  Control_signal_servos : Inport
  Control split : Subsystem  TreatAsAtomicUnit=on
  Mux : Mux  Inputs=[1,1,1,1,1,1,4]
  Mux1 : Mux  Inputs=2
  Selector : Selector  InputPortWidth=3
  Selector1 : Selector  InputPortWidth=3  Indices=2
  Selector2 : Selector  InputPortWidth=3  Indices=3
  Selector3 : Selector  InputPortWidth=7  Indices=[1]
  Selector4 : Selector  InputPortWidth=7  Indices=2
  Selector5 : Selector  InputPortWidth=7  Indices=3
  Selector6 : Selector  InputPortWidth=7  Indices=[4:7]
  r2d : Gain  Gain=180/pi
  r2d1 : Gain  Gain=180/pi
  "Control_signals_serv_deg " : Outport
  wires:
  Mux/1 -> "Control_signals_serv_deg "/1
  Control_signal_servos/1 -> Control split/1(Control inputs)
  Control split/3(Sups control) -> r2d1/1
  Control split/2(Angles) -> r2d/1
  Control split/1("Throtles ") -> Selector1/1, Selector/1, Selector2/1
  Selector/1 -> Mux/1
  Mux1/1 -> Selector5/1, Selector4/1, Selector3/1, Selector6/1
  Selector3/1 -> Mux/2
  Selector1/1 -> Mux/3
  Selector4/1 -> Mux/4
  Selector2/1 -> Mux/5
  Selector5/1 -> Mux/6
  Selector6/1 -> Mux/7
  r2d/1 -> Mux1/1  "Angles_arms"
  r2d1/1 -> Mux1/2  "sups_control"

== system DBX_control_harness/DBX FCS/PWM Interface out ==
  PWM1 : Inport
  PWM2 : Inport  Port=2
  PWM3 : Inport  Port=3
  PWM4 : Inport  Port=4
  PWM5 : Inport  Port=5
  PWM6 : Inport  Port=6
  PWM7 : Inport  Port=7
  PWM8 : Inport  Port=8
  PWM Interface out: Agosto prototipo : Subsystem  TreatAsAtomicUnit=on  VariantControl=Agosto
  PWM Interface out: VTOL : Subsystem  TreatAsAtomicUnit=on  VariantControl=Octubre
  Motores : Outport
  Servos : Outport  Port=2

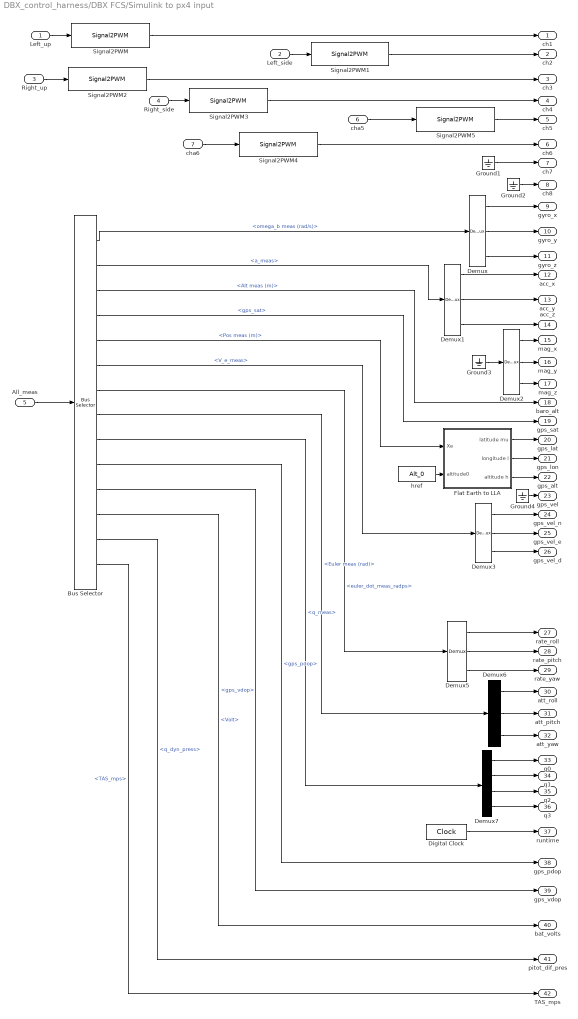
== system DBX_control_harness/DBX FCS/Simulink to px4 input ==
  Left_up : Inport
  Left_side : Inport  Port=2
  Right_up : Inport  Port=3
  Right_side : Inport  Port=4
  All_meas : Inport  Port=5
  cha5 : Inport  Port=6
  cha6 : Inport  Port=7
  Bus Selector : BusSelector  OutputSignals=Meas.omega_b meas (rad/s),Params.a_meas,Meas.Alt meas (m),Params.gps_sat,Meas.Pos meas (m),Meas.V_e_meas,Meas.euler_dot_meas_radps,Meas.Euler meas (rad),Meas.q_meas,Params.gps_pdop,Params.gps_vdop,Meas.Volt,Meas.q_dyn_press,Params.TAS_mps
  Demux{,1..3,5..6} (6 alike) : Demux  Outputs=3
  Demux7 : Demux
  Digital Clock : DigitalClock  SampleTime=T_ctrl
  Flat Earth to LLA : Subsystem
  Ground{1..4} (4 alike) : Ground
  Signal2PWM{,1..5} (6 alike) : DBX_model/Signal2PWM  b=1  d=-1  a=2000  c=1000
  href : Constant  Value=Alt_0  VectorParams1D=off
  ch1 : Outport
  ch2 : Outport  Port=2
  ch3 : Outport  Port=3
  ch4 : Outport  Port=4
  ch5 : Outport  Port=5
  ch6 : Outport  Port=6
  ch7 : Outport  Port=7
  ch8 : Outport  Port=8
  gyro_x : Outport  Port=9
  gyro_y : Outport  Port=10
  gyro_z : Outport  Port=11
  acc_x : Outport  Port=12
  acc_y : Outport  Port=13
  acc_z : Outport  Port=14
  mag_x : Outport  Port=15
  mag_y : Outport  Port=16
  mag_z : Outport  Port=17
  baro_alt : Outport  Port=18
  gps_sat : Outport  Port=19
  gps_lat : Outport  Port=20
  gps_lon : Outport  Port=21
  gps_alt : Outport  Port=22
  gps_vel : Outport  Port=23
  gps_vel_n : Outport  Port=24
  gps_vel_e : Outport  Port=25
  gps_vel_d : Outport  Port=26
  rate_roll : Outport  Port=27
  rate_pitch : Outport  Port=28
  rate_yaw : Outport  Port=29
  att_roll : Outport  Port=30
  att_pitch : Outport  Port=31
  att_yaw : Outport  Port=32
  q0 : Outport  Port=33
  q1 : Outport  Port=34
  q2 : Outport  Port=35
  q3 : Outport  Port=36
  runtime : Outport  Port=37
  gps_pdop : Outport  Port=38
  gps_vdop : Outport  Port=39
  bat_volts : Outport  Port=40
  pitot_dif_pres : Outport  Port=41
  TAS_mps : Outport  Port=42
  wires:
  Left_up/1 -> Signal2PWM/1
  Left_side/1 -> Signal2PWM1/1
  Right_up/1 -> Signal2PWM2/1
  Right_side/1 -> Signal2PWM3/1
  cha6/1 -> Signal2PWM4/1
  Ground1/1 -> ch7/1
  Ground2/1 -> ch8/1
  All_meas/1 -> Bus Selector/1
  href/1 -> Flat Earth to LLA/2(altitude0)
  Demux/1 -> gyro_x/1
  Demux/2 -> gyro_y/1
  Demux/3 -> gyro_z/1
  Bus Selector/1 -> Demux/1  "<omega_b meas (rad/s)>"
  Demux1/1 -> acc_x/1
  Demux1/2 -> acc_y/1
  Demux1/3 -> acc_z/1
  Bus Selector/2 -> Demux1/1  "<a_meas>"
  Ground3/1 -> Demux2/1
  Demux2/1 -> mag_x/1
  Demux2/2 -> mag_y/1
  Demux2/3 -> mag_z/1
  Bus Selector/3 -> baro_alt/1  "<Alt meas (m)>"
  Bus Selector/4 -> gps_sat/1  "<gps_sat>"
  Flat Earth to LLA/1(latitude mu) -> gps_lat/1
  Flat Earth to LLA/2(longitude l) -> gps_lon/1
  Flat Earth to LLA/3(altitude h) -> gps_alt/1
  Bus Selector/5 -> Flat Earth to LLA/1(Xe)  "<Pos meas (m)>"
  Ground4/1 -> gps_vel/1
  Demux3/1 -> gps_vel_n/1
  Demux3/3 -> gps_vel_d/1
  Bus Selector/6 -> Demux3/1  "<V_e_meas>"
  Demux3/2 -> gps_vel_e/1
  Demux5/1 -> rate_roll/1
  Demux5/2 -> rate_pitch/1
  Demux5/3 -> rate_yaw/1
  Demux6/1 -> att_roll/1
  Demux6/2 -> att_pitch/1
  Demux6/3 -> att_yaw/1
  Bus Selector/8 -> Demux6/1  "<Euler meas (rad)>"
  Demux7/1 -> q0/1
  Demux7/2 -> q1/1
  Demux7/3 -> q2/1
  Demux7/4 -> q3/1
  Bus Selector/9 -> Demux7/1  "<q_meas>"
  Bus Selector/10 -> gps_pdop/1  "<gps_pdop>"
  Bus Selector/11 -> gps_vdop/1  "<gps_vdop>"
  Bus Selector/12 -> bat_volts/1  "<Volt>"
  Signal2PWM/1 -> ch1/1
  Signal2PWM1/1 -> ch2/1
  Signal2PWM2/1 -> ch3/1
  Signal2PWM3/1 -> ch4/1
  Digital Clock/1 -> runtime/1
  cha5/1 -> Signal2PWM5/1
  Signal2PWM5/1 -> ch5/1
  Signal2PWM4/1 -> ch6/1
  Bus Selector/13 -> pitot_dif_pres/1  "<q_dyn_press>"
  Bus Selector/14 -> TAS_mps/1  "<TAS_mps>"
  Bus Selector/7 -> Demux5/1  "<euler_dot_meas_radps>"

== system DBX_control_harness/FlightGear visualization/Flat Earth to LLA ==
  note: Flat Earth to LLA
  Xe : Inport
  altitude0 : Inport  Port=2
  Add : Sum
  Demux2 : Demux  Outputs=2
  Mux : Mux  Inputs=2
  Selector : Selector  InputPortWidth=3  Indices=3
  Unary Minus : UnaryMinus
  deg2rad : Gain  Gain=pi/180  SaturateOnIntegerOverflow=on  OutDataTypeStr=Inherit: Same as input  ParamDataTypeStr=Inherit: Same as input
  ne to lat/long : Subsystem
  longitude l : Outport
  latitude mu : Outport  Port=2
  altitude h : Outport  Port=3
  wires:
  Demux2/1 -> latitude mu/1  "latitude"
  Demux2/2 -> longitude l/1
  deg2rad/1 -> Demux2/1
  ne to lat/long/1(lat_deg) -> Mux/1
  ne to lat/long/2(long_deg) -> Mux/2
  Mux/1 -> deg2rad/1
  Selector/1 -> Unary Minus/1
  Add/1 -> altitude h/1
  altitude0/1 -> Add/2
  Xe/1 -> ne to lat/long/1(Xe), Selector/1
  Unary Minus/1 -> Add/1

== system DBX_control_harness/FlightGear visualization/keep pi//pi ==
  phi theta psi : Inport
  Constant : Constant  Value=180
  Constant2 : Constant  Value=360
  Gain : Gain  Gain=360
  Math Function2 : Math  Operator=rem  SaturateOnIntegerOverflow=on
  Product : Product  Inputs=*/  RndMeth=Zero
  Rounding Function : Rounding  Operator=fix
  Sum2 : Sum  Inputs=|-+
  deg2rad1 : Gain  Gain=pi/180  SaturateOnIntegerOverflow=on  OutDataTypeStr=Inherit: Same as input  ParamDataTypeStr=Inherit: Same as input
  rad2deg : Gain  Gain=180/pi  SaturateOnIntegerOverflow=on  OutDataTypeStr=Inherit: Same as input  ParamDataTypeStr=Inherit: Same as input
  ptp_earth : Outport
  wires:
  phi theta psi/1 -> rad2deg/1
  Constant/1 -> Product/2
  Product/1 -> Rounding Function/1
  Rounding Function/1 -> Gain/1
  Gain/1 -> Sum2/1
  rad2deg/1 -> Math Function2/1
  Constant2/1 -> Math Function2/2
  Math Function2/1 -> Product/1, Sum2/2
  Sum2/1 -> deg2rad1/1
  deg2rad1/1 -> ptp_earth/1

== system DBX_control_harness/Parameters estimation/DCM1 ==
  Euler : Inport  PortDimensions=3
  Fcn11 : Fcn  Expr=u(5)*u(4)
  Fcn12 : Fcn  Expr=u(5)*u(1)
  Fcn13 : Fcn  Expr=-u(2)
  Fcn21 : Fcn  Expr=u(3)*u(2)*u(4) - u(6)*u(1)
  Fcn22 : Fcn  Expr=u(3)*u(2)*u(1) + u(6)*u(4)
  Fcn23 : Fcn  Expr=u(3)*u(5)
  Fcn31 : Fcn  Expr=u(6)*u(2)*u(4) + u(3)*u(1)
  Fcn32 : Fcn  Expr=u(6)*u(2)*u(1) - u(3)*u(4)
  Fcn33 : Fcn  Expr=u(6)*u(5)
  Mux : Mux  Inputs=2
  Mux1 : Mux  Inputs=9
  Reshape : Reshape  OutputDimensionality=Customize  OutputDimensions=[3,3]
  sincos : Trigonometry  Operator=sincos
  DCM : Outport  PortDimensions=[3,3]
  wires:
  Fcn33/1 -> Mux1/9
  Fcn32/1 -> Mux1/8
  Fcn23/1 -> Mux1/6
  Fcn22/1 -> Mux1/5
  Fcn31/1 -> Mux1/7
  Fcn21/1 -> Mux1/4
  Fcn13/1 -> Mux1/3
  Fcn12/1 -> Mux1/2
  Fcn11/1 -> Mux1/1
  Mux/1 -> Fcn22/1, Fcn23/1, Fcn31/1, Fcn33/1, Fcn32/1, Fcn21/1, Fcn13/1, Fcn12/1, Fcn11/1
  sincos/2 -> Mux/2
  sincos/1 -> Mux/1
  Reshape/1 -> DCM/1
  Euler/1 -> sincos/1
  Mux1/1 -> Reshape/1

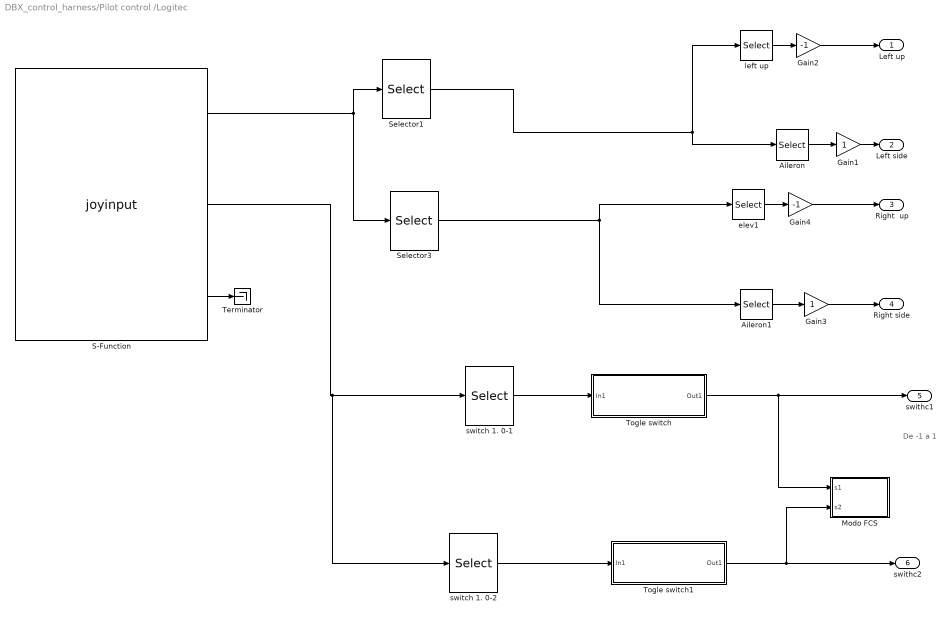
== system DBX_control_harness/Pilot control /Logitec  ==
  note: De -1 a 1
  Aileron : Selector  InputPortWidth=2
  Aileron1 : Selector  InputPortWidth=2
  Gain1 : Gain
  Gain2 : Gain  Gain=-1
  Gain3 : Gain
  Gain4 : Gain  Gain=-1
  Modo FCS : MATLAB Function  TreatAsAtomicUnit=on
  S-Function : S-Function  FunctionName=joyinput  Parameters=joyid,adjustports,forcefeed  mask{joyid=1, adjustports=on, forcefeed=off}
      mask prompts: joyid "Joystick ID:"; adjustports "Adjust ports?"; forcefeed "Enable force"
      mask init:
      | label = 'image(imread(''joystickicon.png'')); port_label(''output'', 1, ''Axes''); port_label(''output'', 2, ''Buttons''); ';
      | porthandles = get_param(gcbh, 'PortHandles');
      | if numel(porthandles.Outport)>2
      |   label = [label 'port_label(''output'', 3, ''Point of View''); '];
      | end
      | if numel(porthandles.Inport)>0  label = [label 'port_label(''input'', 1, ''Force''); '];
      | end
      | set_param(gcbh, 'MaskDisplay', label);
      mask Help: helpview(vrmfunc('FnHelpTopic'), 'vr_joystickinput');
      mask Display: image(imread('joystickicon.png')); port_label('output', 1, 'Axes'); port_label('output', 2, 'Buttons'); port_label('output', 3, 'Point of View');
  Selector1 : Selector  InputPortWidth=5  Indices=1:2
  Selector3 : Selector  InputPortWidth=5  Indices=4:5
  Terminator : Terminator
  Togle switch : Subsystem
  Togle switch1 : Subsystem
  elev1 : Selector  InputPortWidth=2  Indices=2
  left up : Selector  InputPortWidth=2  Indices=2
  switch 1. 0-1 : Selector  InputPortWidth=10  Indices=5
  switch 1. 0-2 : Selector  InputPortWidth=10  Indices=6
  Left up : Outport
  Left side : Outport  Port=2
  Right  up : Outport  Port=3
  Right side : Outport  Port=4
  swithc1 : Outport  Port=5
  swithc2 : Outport  Port=6
  wires:
  switch 1. 0-2/1 -> Togle switch1/1(In1)
  Togle switch/1(Out1) -> Modo FCS/1(s1), swithc1/1
  switch 1. 0-1/1 -> Togle switch/1(In1)
  S-Function/2 -> switch 1. 0-1/1, switch 1. 0-2/1
  Gain2/1 -> Left up/1
  Togle switch1/1(Out1) -> Modo FCS/2(s2), swithc2/1
  Selector3/1 -> elev1/1, Aileron1/1
  Gain4/1 -> Right  up/1
  Gain3/1 -> Right side/1
  elev1/1 -> Gain4/1
  Aileron1/1 -> Gain3/1
  S-Function/3 -> Terminator/1
  Gain1/1 -> Left side/1
  left up/1 -> Gain2/1
  S-Function/1 -> Selector3/1, Selector1/1
  Selector1/1 -> left up/1, Aileron/1
  Aileron/1 -> Gain1/1

== system DBX_control_harness/Pilot control /Signal generator ==
  Constant : Constant
  Constant1 : Constant  Value=-0.1
  Signal Builder : Subsystem  Tag=STV Subsys  LoadFcn=sigbuilder_block('load');  StartFcn=sigbuilder_block('start');  StopFcn=sigbuilder_block('stop');  ClipboardFcn=sigbuilder_block('clipboard');  mask(Sigbuilder block){}
      mask help: Simulink:masks:SigbuilderBlock_MD
      mask init:
      | if ~strcmp(get_param(bdroot(gcbh),'SimulationStatus'),'stopped') tuvar = sigbuilder_block('maskInit'); end
      settings: CopyFcn=sigbuilder_block('copy');  DeleteFcn=sigbuilder_block('delete');  ModelCloseFcn=sigbuilder_block('modelClose');  PreSaveFcn=sigbuilder_block('preSave');  PauseFcn=sigbuilder_block('pause');  ContinueFcn=sigbuilder_block('continue');  NameChangeFcn=sigbuilder_block('namechange');  OpenFcn=sigbuilder_block('open',[437.6 199.2 550.4 400 ]);  CloseFcn=sigbuilder_block('close');
      mask Display: plot(0, 0, 100, 100,[2, 2, 32, 32, 2], [68, 8, 8, 68, 68],[32, 2], [38, 38], [32, 19, 2],[53, 60, 44], [32, 17, 17, 2],[16, 16, 31, 31]);txt = getActiveGroup(gcbh);text(2, 100, txt,'verticalAlignment', 'top');
  Unit Delay : UnitDelay  InitialCondition=-1  SampleTime=-1
  Unit Delay1 : UnitDelay  InitialCondition=-1  SampleTime=-1
  Left up : Outport
  Left side : Outport  Port=2
  Right  up : Outport  Port=3
  Right side : Outport  Port=4
  swithc1 : Outport  Port=5
  swithc2 : Outport  Port=6
  wires:
  Unit Delay/1 -> Unit Delay1/1, swithc1/1
  Constant/1 -> Unit Delay/1
  Unit Delay1/1 -> swithc2/1
  Signal Builder/2(Signal 2) -> Right side/1
  Signal Builder/1(Signal 1) -> Right  up/1
  Constant1/1 -> Left up/1

== system DBX_control_harness/Pilot control /Turnigy TX (XTR G2 FMS) ==
  note: De -1 a 1
  Bias : Bias  Bias=-1
  Demux : Demux  Outputs=6
  Display2 : Display
  Gain : Gain  Gain=2  OutDataTypeStr=double
  S-Function : S-Function  FunctionName=joyinput  Parameters=joyid,adjustports,forcefeed  mask{joyid=1, adjustports=on, forcefeed=off}
      mask prompts: joyid "Joystick ID:"; adjustports "Adjust ports?"; forcefeed "Enable force"
      mask init: same as DBX_control_harness/Pilot control /Logitec /S-Function
      mask Help: helpview(vrmfunc('FnHelpTopic'), 'vr_joystickinput');
      mask Display: image(imread('joystickicon.png')); port_label('output', 1, 'Axes'); port_label('output', 2, 'Buttons');
  Selector6 : Selector  InputPortWidth=4
  Terminator : Terminator
  Left up : Outport
  Left side : Outport  Port=2
  Right  up : Outport  Port=3
  Right side : Outport  Port=4
  swithc1 : Outport  Port=5
  swithc2 : Outport  Port=6
  wires:
  S-Function/2 -> Selector6/1
  Demux/2 -> Left up/1
  Demux/4 -> Left side/1
  Demux/1 -> Right  up/1
  Demux/5 -> Right side/1
  Demux/6 -> swithc2/1
  Demux/3 -> Terminator/1
  S-Function/1 -> Display2/1, Demux/1
  Selector6/1 -> Gain/1
  Gain/1 -> Bias/1
  Bias/1 -> swithc1/1

== system DBX_control_harness/Plotting/Deflex mixer ==
  note: Control inputs:
      |
      |
      | 7. Rudervator Left (rad)
      | 8. Rudervator Right (rad)
      | 9. Aileron Left (rad)
      | 10. Aielron Right (rad)
  Sups_control : Inport
  Add : Sum  Inputs=|+-
  Add1 : Sum  Inputs=|++
  Add2 : Sum  Inputs=|+-
  Demux : Demux
  Gain : Gain  Gain=1/2
  Gain1 : Gain  Gain=1/2
  Gain2 : Gain  Gain=1/2
  delta_ail_Asim : Outport
  delta_rv_sim : Outport  Port=2
  delta_rv_Asim : Outport  Port=3
  wires:
  Sups_control/1 -> Demux/1
  Demux/3 -> Add/1
  Demux/4 -> Add/2
  Add/1 -> Gain/1
  Gain/1 -> delta_ail_Asim/1
  Demux/1 -> Add2/1, Add1/1
  Demux/2 -> Add2/2, Add1/2
  Add2/1 -> Gain1/1
  Add1/1 -> Gain2/1
  Gain2/1 -> delta_rv_sim/1
  Gain1/1 -> delta_rv_Asim/1

== system DBX_control_harness/Plotting/Deflex mixer1 ==
  note: Control inputs:
      |
      |
      | 7. Rudervator Left (rad)
      | 8. Rudervator Right (rad)
      | 9. Aileron Left (rad)
      | 10. Aielron Right (rad)
  Sups_control : Inport
  Add : Sum  Inputs=|+-
  Add1 : Sum  Inputs=|++
  Add2 : Sum  Inputs=|+-
  Demux : Demux
  Gain : Gain  Gain=1/2
  Gain1 : Gain  Gain=1/2
  Gain2 : Gain  Gain=1/2
  delta_ail_Asim : Outport
  delta_rv_sim : Outport  Port=2
  delta_rv_Asim : Outport  Port=3
  wires:
  Gain1/1 -> delta_rv_Asim/1
  Gain2/1 -> delta_rv_sim/1
  Add1/1 -> Gain2/1
  Add2/1 -> Gain1/1
  Demux/2 -> Add1/2, Add2/2
  Demux/1 -> Add1/1, Add2/1
  Gain/1 -> delta_ail_Asim/1
  Add/1 -> Gain/1
  Demux/4 -> Add/2
  Demux/3 -> Add/1
  Sups_control/1 -> Demux/1

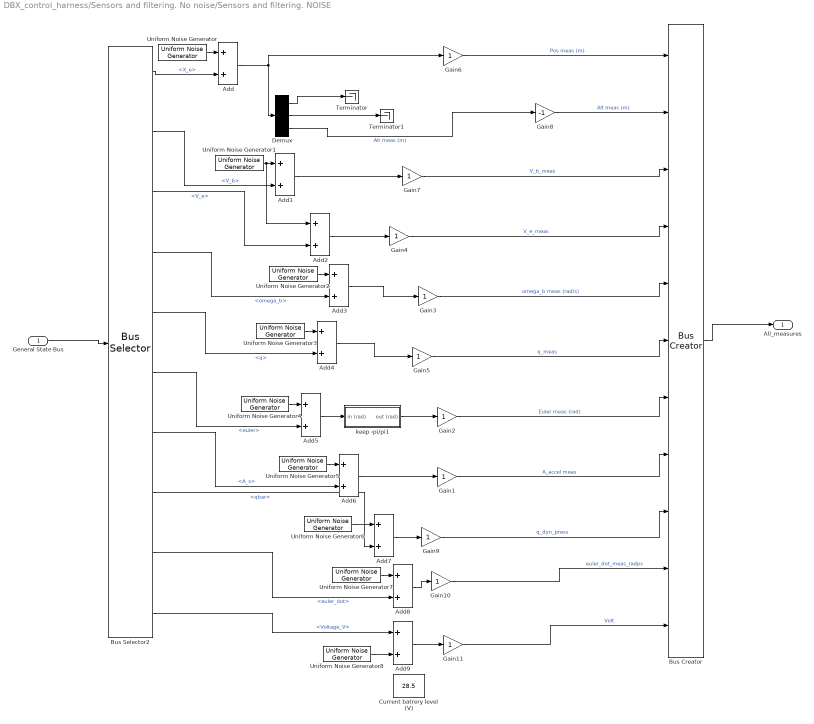
== system DBX_control_harness/Sensors and filtering. No noise/Sensors and filtering. NOISE ==
  General State Bus : Inport
  Add{,1..9} (10 alike) : Sum
  Bus Creator : BusCreator  Inputs=11
  Bus Selector2 : BusSelector  OutputSignals=X_e,V_b,V_e,omega_b,q,euler,A_s,Aero_vars.qbar,euler_dot,Battery_bus.Voltage_V
  Current batrery level (V) : Constant  Value=28.5
  Demux : Demux  Outputs=3
  Gain{1..7,9..11} (10 alike) : Gain
  Gain8 : Gain  Gain=-1
  Terminator : Terminator
  Terminator1 : Terminator
  Uniform Noise Generator : commnoisgen2/Uniform Noise Generator  low=-GPS_pos_sig*[1,1,1]'  up=GPS_pos_sig*[1,1,1]'  seed=31  Ts=T_sim  frameBased=off  sampPerFrame=1  orient=off  outDataType=double
  Uniform Noise Generator1 : commnoisgen2/Uniform Noise Generator  low=-Speed_sigmas*[1,1,1]'  up=Speed_sigmas*[1,1,1]'  seed=35  Ts=T_sim  frameBased=off  sampPerFrame=1  orient=off  outDataType=double
  Uniform Noise Generator2 : commnoisgen2/Uniform Noise Generator  low=-omgea_b_sigmas*[1,1,1]'  up=omgea_b_sigmas*[1,1,1]'  seed=2  Ts=T_sim  frameBased=off  sampPerFrame=1  orient=off  outDataType=double
  Uniform Noise Generator3 : commnoisgen2/Uniform Noise Generator  low=-quaternion_sigmas*[1,1,1,1]'  up=quaternion_sigmas*[1,1,1,1]'  seed=12  Ts=T_sim  frameBased=off  sampPerFrame=1  orient=off  outDataType=double
  Uniform Noise Generator4 : commnoisgen2/Uniform Noise Generator  low=-Euler_sigmas*[1,1,10]'  up=Euler_sigmas*[1,1,10]'  seed=69  Ts=T_sim  frameBased=off  sampPerFrame=1  orient=off  outDataType=double
  Uniform Noise Generator5 : commnoisgen2/Uniform Noise Generator  low=-accel_sigmas*[1,1,1]'  up=accel_sigmas*[1,1,1]'  seed=62  Ts=T_sim  frameBased=off  sampPerFrame=1  orient=off  outDataType=double
  Uniform Noise Generator6 : commnoisgen2/Uniform Noise Generator  low=-qbar_sigma  up=qbar_sigma  seed=56  Ts=T_sim  frameBased=off  sampPerFrame=1  orient=off  outDataType=double
  Uniform Noise Generator7 : commnoisgen2/Uniform Noise Generator  low=-Euler_dot_sigmas*[1,1,1]'  up=Euler_dot_sigmas*[1,1,1]'  seed=69  Ts=T_sim  frameBased=off  sampPerFrame=1  orient=off  outDataType=double
  Uniform Noise Generator8 : commnoisgen2/Uniform Noise Generator  low=-Volt_noise  up=Volt_noise  seed=33  Ts=T_sim  frameBased=off  sampPerFrame=1  orient=off  outDataType=double
  keep -pi/pi1 : Subsystem
  All_measures : Outport
  wires:
  Gain10/1 -> Bus Creator/10  "euler_dot_meas_radps"
  Gain9/1 -> Bus Creator/9  "q_dyn_press"
  Bus Selector2/8 -> Add7/2  "<qbar>"
  Gain11/1 -> Bus Creator/11  "Volt"
  General State Bus/1 -> Bus Selector2/1
  Bus Selector2/1 -> Add/2  "<X_e>"
  Gain8/1 -> Bus Creator/2  "Alt meas (m)"
  Demux/1 -> Terminator/1
  Demux/2 -> Terminator1/1
  Gain7/1 -> Bus Creator/3  "V_b_meas"
  Gain3/1 -> Bus Creator/5  "omega_b meas (rad/s)"
  Bus Creator/1 -> All_measures/1
  Demux/3 -> Gain8/1  "Alt meas (m)"
  Gain2/1 -> Bus Creator/7  "Euler meas (rad)"
  Gain1/1 -> Bus Creator/8  "A_accel meas"
  Bus Selector2/3 -> Add2/2  "<V_e>"
  Gain4/1 -> Bus Creator/4  "V_e_meas"
  Gain5/1 -> Bus Creator/6  "q_meas"
  Gain6/1 -> Bus Creator/1  "Pos meas (m)"
  keep -pi/pi1/1(out (rad)) -> Gain2/1
  Uniform Noise Generator/1 -> Add/1
  Add/1 -> Demux/1, Gain6/1
  Uniform Noise Generator1/1 -> Add2/1, Add1/1
  Bus Selector2/2 -> Add1/2  "<V_b>"
  Add1/1 -> Gain7/1
  Add2/1 -> Gain4/1
  Uniform Noise Generator2/1 -> Add3/1
  Add3/1 -> Gain3/1
  Bus Selector2/4 -> Add3/2  "<omega_b>"
  Uniform Noise Generator3/1 -> Add4/1
  Add4/1 -> Gain5/1
  Bus Selector2/5 -> Add4/2  "<q>"
  Uniform Noise Generator4/1 -> Add5/1
  Add5/1 -> keep -pi/pi1/1(in (rad))
  Bus Selector2/6 -> Add5/2  "<euler>"
  Add6/1 -> Gain1/1
  Uniform Noise Generator5/1 -> Add6/1
  Bus Selector2/7 -> Add6/2  "<A_s>"
  Uniform Noise Generator6/1 -> Add7/1
  Add7/1 -> Gain9/1
  Add8/1 -> Gain10/1
  Uniform Noise Generator7/1 -> Add8/1
  Bus Selector2/9 -> Add8/2  "<euler_dot>"
  Add9/1 -> Gain11/1
  Bus Selector2/10 -> Add9/1  "<Voltage_V>"
  Uniform Noise Generator8/1 -> Add9/2

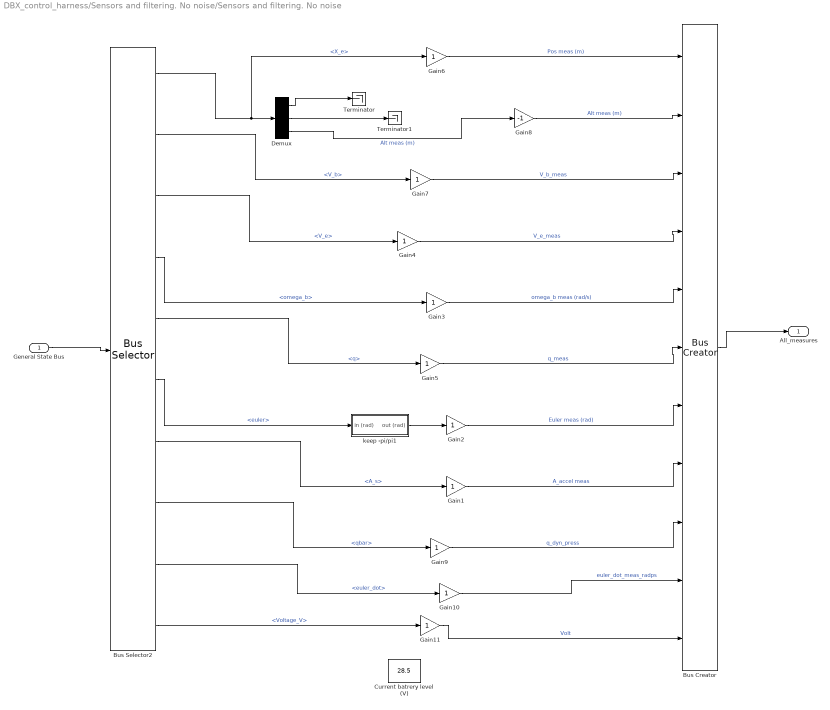
== system DBX_control_harness/Sensors and filtering. No noise/Sensors and filtering. No noise ==
  General State Bus : Inport
  Bus Creator : BusCreator  Inputs=11
  Bus Selector2 : BusSelector  OutputSignals=X_e,V_b,V_e,omega_b,q,euler,A_s,Aero_vars.qbar,euler_dot,Battery_bus.Voltage_V
  Current batrery level (V) : Constant  Value=28.5
  Demux : Demux  Outputs=3
  Gain{1..7,9..11} (10 alike) : Gain
  Gain8 : Gain  Gain=-1
  Terminator : Terminator
  Terminator1 : Terminator
  keep -pi/pi1 : Subsystem
  All_measures : Outport
  wires:
  keep -pi/pi1/1(out (rad)) -> Gain2/1
  Gain6/1 -> Bus Creator/1  "Pos meas (m)"
  Gain5/1 -> Bus Creator/6  "q_meas"
  Bus Selector2/5 -> Gain5/1  "<q>"
  Gain4/1 -> Bus Creator/4  "V_e_meas"
  Bus Selector2/3 -> Gain4/1  "<V_e>"
  Gain1/1 -> Bus Creator/8  "A_accel meas"
  Bus Selector2/7 -> Gain1/1  "<A_s>"
  Gain2/1 -> Bus Creator/7  "Euler meas (rad)"
  Demux/3 -> Gain8/1  "Alt meas (m)"
  Bus Creator/1 -> All_measures/1
  Gain3/1 -> Bus Creator/5  "omega_b meas (rad/s)"
  Gain7/1 -> Bus Creator/3  "V_b_meas"
  Bus Selector2/6 -> keep -pi/pi1/1(in (rad))  "<euler>"
  Bus Selector2/4 -> Gain3/1  "<omega_b>"
  Bus Selector2/2 -> Gain7/1  "<V_b>"
  Demux/2 -> Terminator1/1
  Demux/1 -> Terminator/1
  Gain8/1 -> Bus Creator/2  "Alt meas (m)"
  Bus Selector2/1 -> Demux/1, Gain6/1  "<X_e>"
  General State Bus/1 -> Bus Selector2/1
  Gain11/1 -> Bus Creator/11  "Volt"
  Bus Selector2/8 -> Gain9/1  "<qbar>"
  Gain9/1 -> Bus Creator/9  "q_dyn_press"
  Bus Selector2/9 -> Gain10/1  "<euler_dot>"
  Gain10/1 -> Bus Creator/10  "euler_dot_meas_radps"
  Bus Selector2/10 -> Gain11/1  "<Voltage_V>"

== system DBX_control_harness/Signals reality/PWM resolution ==
  PWM_us in : Inport
  Quantizer : Quantizer  QuantizationInterval=DBX_PWM.quant_interval
  PWM_us out : Outport
  wires:
  PWM_us in/1 -> Quantizer/1
  Quantizer/1 -> PWM_us out/1

== system DBX_control_harness/Signals reality/PWM resolution1 ==
  PWM_us in : Inport
  Quantizer : Quantizer  QuantizationInterval=DBX_PWM.quant_interval
  PWM_us out : Outport
  wires:
  Quantizer/1 -> PWM_us out/1
  PWM_us in/1 -> Quantizer/1

== system DBX_control_harness/Signals reality/Re-Build Signals servos ==
  note: Control inputs (Servos angles in rads):
      | 2. eta_1 (rad)  (Pan arm 1)
      |
      | 4. eta_2 (rad)  (Pan arm 2)
      |
      | 6. eta_3 (rad)  (Pan arm  3)
      |
      | 7. Rudervator Left (rad)
      | 8. Rudervator Right (rad)
      | 9. Aileron Left (rad)
      | 10. Aielron Right (rad)
  PWM_us servos in : Inport
  Demux : Demux  Outputs=7
  Mux : Mux  Inputs=7
  PWM2signal{,1..6} (7 alike) : DBX_model/PWM2signal  c=DBX_PWM.Servos.Max_PWM  a=DBX_PWM.Servos.Min_PWM  d=deg2rad(90)  b=-deg2rad(90)
  signals out : Outport
  wires:
  PWM_us servos in/1 -> Demux/1
  Demux/6 -> PWM2signal1/1
  Demux/5 -> PWM2signal2/1
  Demux/4 -> PWM2signal3/1
  Demux/3 -> PWM2signal4/1
  Demux/2 -> PWM2signal5/1
  Demux/1 -> PWM2signal6/1
  PWM2signal6/1 -> Mux/1
  PWM2signal5/1 -> Mux/2
  PWM2signal3/1 -> Mux/4
  PWM2signal2/1 -> Mux/5
  Mux/1 -> signals out/1
  PWM2signal4/1 -> Mux/3
  PWM2signal1/1 -> Mux/6
  Demux/7 -> PWM2signal/1
  PWM2signal/1 -> Mux/7

== system DBX_control_harness/rad2deg1/Control split ==
  Control inputs : Inport
  Throttles : Selector  InputPortWidth=10  Indices=[1,3,5]
  Throttles1 : Selector  InputPortWidth=10  Indices=[2,4,6]
  Throttles2 : Selector  InputPortWidth=10  Indices=[7:10]
  "Throtles " : Outport
  Angles : Outport  Port=2
  Sups control : Outport  Port=3
  wires:
  Control inputs/1 -> Throttles2/1, Throttles1/1, Throttles/1
  Throttles1/1 -> Angles/1
  Throttles/1 -> "Throtles "/1
  Throttles2/1 -> Sups control/1
